simulink model "Model_InterpretationEngine64"  (R2022b)
settings: Solver=FixedStepDiscrete  StartTime=0.0  StopTime=5  RelTol=1e-3  EnableMultiTasking=on
InitFcn:
  | % Initialize model
  | ModelSettings=BTConfig.GetModelSettings();
  | 
  | ModelSettings.Validate();
  | 
  | ModelInit;
  | 
  | 
  | % load library data
  | GainLibrary_data;
  | % Load saved values from partition process
  | CapturedConstMask.LoadMapFromFile(bdroot)
  | % Load saved values from partition process
  | TSP_Mask.LoadMapFromFile(bdroot)
StartFcn:
  | % make sure all the simulated RTC requests are found
  | %RTC_SIM_OBJ.ValidateREQs();
undefined symbols (not defined in the file or in its folder): NumHFRefBPF, NumHFRefLPF
libraries: StateVar x112, TSP x56, FeaturePath x24
(part 3 of 5)

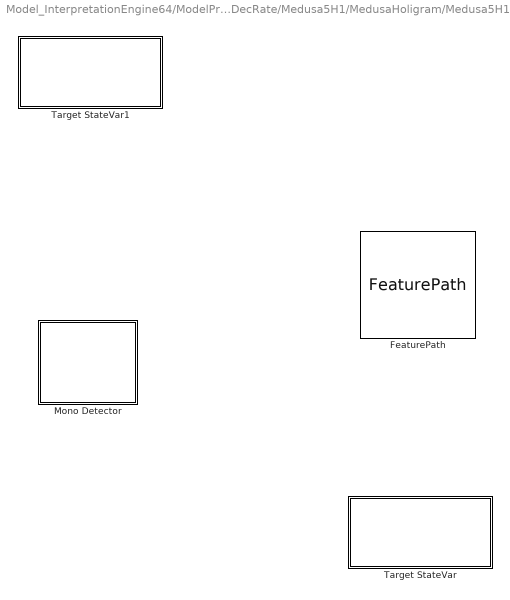
== system Model_InterpretationEngine64/ModelPreAmp/DecRate/Medusa5H1/MedusaHoligram/Medusa5H1 Part 2/Mono Detector ==
  FeaturePath : FeaturePath/FeaturePath  FeatureName=MonoDetector  IsGroup=off  GroupNumber=-1  IsModule=off  TriggerInit=[680 129 795 236]
      settings: SourceProductName=Bose Talaria
  Mono Detector : Subsystem
  Target StateVar : Subsystem  mask(Talaria Target State Variable){TriggerInit=[670 396 810 464], TspName=IsStereo, StateName=IsStereo, UseSameName=on, IfdefMacro=[]}
      mask prompts: TriggerInit "Hidden: MoveFcn redraw"; TspName "Name:"; StateName "Name of StateVar:"; UseSameName "Use same name for state variable and TSP"; IfdefMacro "Additional #ifdef macro to enable trigger capture:"
      mask help: The TargetStateVar block encapsultes a Target State Probe (TSP), a State Variable, and a Trivial Interpretation between them.
      mask init:
      | [ok,tspPath,activeStatePath] = TargetStateVarMask.Init(gcbh);
      settings: MoveFcn=TargetStateVarMask.CB_TriggerInit(gcbh);
      mask Help: See help for StateVar and TSP blocks
      mask Callback TriggerInit: TargetStateVarMask.CB_TriggerInit(gcbh);
      mask TypeOptions TspName: TSP/TspName
      mask TypeOptions StateName: StateVar/StateName
      mask Callback UseSameName: TargetStateVarMask.CB_UseSameName(gcbh);
      mask TypeOptions IfdefMacro: TSP/IfdefMacro
      mask DialogControl AdvancedPanel Prompt: Advanced
      mask DialogControl ConvertToFullInterpretation Prompt: Irreversible conversion to full interpretation
      mask DialogControl ConvertToFullInterpretation Callback: TargetStateVarMask.CB_ConvertToFullInterpretation(gcbh);
      mask DialogControl ErrorContainer Prompt: Error Messages
      mask DialogControl ErrorText Prompt: The interpreted StateVar value is not yet available
      mask DialogControl TspPathText Prompt: TSP: Current parameter name: [PreAmpMedusaMonoDetectorIsStereo]
      mask Display:
      | % retrieve icon definition
      | [path,w,h] = TargetStateVarMask.Icon();
      | 
      | % retrieve the block's pixel size
      | pos = get(gcbh,'position');
      | bw = pos(3) - pos(1);
      | bh = pos(4) - pos(2);
      | 
      | % draw centered icon
      | xAdj = bw/2 - w/2 + 5;
      | yAdj = bh/2 - h/2 + 4;
      | for i=1:length(path)
      | 	patch(path(i).x+xAdj, path(i).y+yAdj, path(i).rgb);
      | end
      | 
      | % show the top name or an X
      | if (exist('ok','var') && ok)
      | 	text(bw*0.5, bh*0.2, tspPath, 'horizontalAlignment', 'center');
      | 	patch(0,0,[1 1 1]);
      | 	patch(bw,bh,[1 1 1]);
      | else
      | 	tx=bw*0.03;
      | 	ty=bh*0.03;
      | 	patch([0 tx bw bw-tx], [ty 0 bh-ty bh], [1 0 0]);
      | 	patch([0 bw-tx bw tx], [bh-ty 0 ty bh], [1 0 0]);
      | end
  Target StateVar1 : Subsystem  mask(Talaria Target State Variable){TriggerInit=[340 131 480 199], TspName=IsActive, StateName=IsActive, UseSameName=on, IfdefMacro=[]}
      mask prompts: TriggerInit "Hidden: MoveFcn redraw"; TspName "Name:"; StateName "Name of StateVar:"; UseSameName "Use same name for state variable and TSP"; IfdefMacro "Additional #ifdef macro to enable trigger capture:"
      mask help: The TargetStateVar block encapsultes a Target State Probe (TSP), a State Variable, and a Trivial Interpretation between them.
      mask init:
      | [ok,tspPath,activeStatePath] = TargetStateVarMask.Init(gcbh);
      settings: MoveFcn=TargetStateVarMask.CB_TriggerInit(gcbh);
      mask Help: See help for StateVar and TSP blocks
      mask Callback TriggerInit: TargetStateVarMask.CB_TriggerInit(gcbh);
      mask TypeOptions TspName: TSP/TspName
      mask TypeOptions StateName: StateVar/StateName
      mask Callback UseSameName: TargetStateVarMask.CB_UseSameName(gcbh);
      mask TypeOptions IfdefMacro: TSP/IfdefMacro
      mask DialogControl AdvancedPanel Prompt: Advanced
      mask DialogControl ConvertToFullInterpretation Prompt: Irreversible conversion to full interpretation
      mask DialogControl ConvertToFullInterpretation Callback: TargetStateVarMask.CB_ConvertToFullInterpretation(gcbh);
      mask DialogControl ErrorContainer Prompt: Error Messages
      mask DialogControl ErrorText Prompt: The interpreted StateVar value is not yet available
      mask DialogControl TspPathText Prompt: TSP: Current parameter name: [PreAmpMedusaMonoDetectorIsActive]
      mask Display:
      | % retrieve icon definition
      | [path,w,h] = TargetStateVarMask.Icon();
      | 
      | % retrieve the block's pixel size
      | pos = get(gcbh,'position');
      | bw = pos(3) - pos(1);
      | bh = pos(4) - pos(2);
      | 
      | % draw centered icon
      | xAdj = bw/2 - w/2 + 5;
      | yAdj = bh/2 - h/2 + 4;
      | for i=1:length(path)
      | 	patch(path(i).x+xAdj, path(i).y+yAdj, path(i).rgb);
      | end
      | 
      | % show the top name or an X
      | if (exist('ok','var') && ok)
      | 	text(bw*0.5, bh*0.2, tspPath, 'horizontalAlignment', 'center');
      | 	patch(0,0,[1 1 1]);
      | 	patch(bw,bh,[1 1 1]);
      | else
      | 	tx=bw*0.03;
      | 	ty=bh*0.03;
      | 	patch([0 tx bw bw-tx], [ty 0 bh-ty bh], [1 0 0]);
      | 	patch([0 bw-tx bw tx], [bh-ty 0 ty bh], [1 0 0]);
      | end

== system Model_InterpretationEngine64/NEAR/Near1p1/VolumeMute/VolMuteCh1/Ann1NonEntGainCalc/boost ==
  Target StateVar : Subsystem  mask(Talaria Target State Variable){TriggerInit=[655 408 850 472], TspName=GetNonEntBoostLeveldB, StateName=GetNonEntBoostLeveldB, UseSameName=on, IfdefMacro=[]}
      mask prompts: TriggerInit "Hidden: MoveFcn redraw"; TspName "Name:"; StateName "Name of StateVar:"; UseSameName "Use same name for state variable and TSP"; IfdefMacro "Additional #ifdef macro to enable trigger capture:"
      mask help: The TargetStateVar block encapsultes a Target State Probe (TSP), a State Variable, and a Trivial Interpretation between them.
      mask init:
      | [ok,tspPath,activeStatePath] = TargetStateVarMask.Init(gcbh);
      settings: MoveFcn=TargetStateVarMask.CB_TriggerInit(gcbh);
      mask Help: See help for StateVar and TSP blocks
      mask Callback TriggerInit: TargetStateVarMask.CB_TriggerInit(gcbh);
      mask TypeOptions TspName: TSP/TspName
      mask TypeOptions StateName: StateVar/StateName
      mask Callback UseSameName: TargetStateVarMask.CB_UseSameName(gcbh);
      mask TypeOptions IfdefMacro: TSP/IfdefMacro
      mask DialogControl AdvancedPanel Prompt: Advanced
      mask DialogControl ConvertToFullInterpretation Prompt: Irreversible conversion to full interpretation
      mask DialogControl ConvertToFullInterpretation Callback: TargetStateVarMask.CB_ConvertToFullInterpretation(gcbh);
      mask DialogControl ErrorContainer Prompt: Error Messages
      mask DialogControl ErrorText Prompt: The interpreted StateVar value is not yet available
      mask DialogControl TspPathText Prompt: TSP: Current parameter name: [NearAnn1Ann1NonEntGainCalcGetNonEntBoostLeveldB]
      mask Display:
      | % retrieve icon definition
      | [path,w,h] = TargetStateVarMask.Icon();
      | 
      | % retrieve the block's pixel size
      | pos = get(gcbh,'position');
      | bw = pos(3) - pos(1);
      | bh = pos(4) - pos(2);
      | 
      | % draw centered icon
      | xAdj = bw/2 - w/2 + 5;
      | yAdj = bh/2 - h/2 + 4;
      | for i=1:length(path)
      | 	patch(path(i).x+xAdj, path(i).y+yAdj, path(i).rgb);
      | end
      | 
      | % show the top name or an X
      | if (exist('ok','var') && ok)
      | 	text(bw*0.5, bh*0.2, tspPath, 'horizontalAlignment', 'center');
      | 	patch(0,0,[1 1 1]);
      | 	patch(bw,bh,[1 1 1]);
      | else
      | 	tx=bw*0.03;
      | 	ty=bh*0.03;
      | 	patch([0 tx bw bw-tx], [ty 0 bh-ty bh], [1 0 0]);
      | 	patch([0 bw-tx bw tx], [bh-ty 0 ty bh], [1 0 0]);
      | end

== system Model_InterpretationEngine64/NEAR/Near1p1/VolumeMute/VolMuteCh2/Ann2NonEntGainCalc/boost ==
  Target StateVar : Subsystem  mask(Talaria Target State Variable){TriggerInit=[655 408 850 472], TspName=GetNonEntBoostLeveldB, StateName=GetNonEntBoostLeveldB, UseSameName=on, IfdefMacro=[]}
      mask prompts: TriggerInit "Hidden: MoveFcn redraw"; TspName "Name:"; StateName "Name of StateVar:"; UseSameName "Use same name for state variable and TSP"; IfdefMacro "Additional #ifdef macro to enable trigger capture:"
      mask help: The TargetStateVar block encapsultes a Target State Probe (TSP), a State Variable, and a Trivial Interpretation between them.
      mask init:
      | [ok,tspPath,activeStatePath] = TargetStateVarMask.Init(gcbh);
      settings: MoveFcn=TargetStateVarMask.CB_TriggerInit(gcbh);
      mask Help: See help for StateVar and TSP blocks
      mask Callback TriggerInit: TargetStateVarMask.CB_TriggerInit(gcbh);
      mask TypeOptions TspName: TSP/TspName
      mask TypeOptions StateName: StateVar/StateName
      mask Callback UseSameName: TargetStateVarMask.CB_UseSameName(gcbh);
      mask TypeOptions IfdefMacro: TSP/IfdefMacro
      mask DialogControl AdvancedPanel Prompt: Advanced
      mask DialogControl ConvertToFullInterpretation Prompt: Irreversible conversion to full interpretation
      mask DialogControl ConvertToFullInterpretation Callback: TargetStateVarMask.CB_ConvertToFullInterpretation(gcbh);
      mask DialogControl ErrorContainer Prompt: Error Messages
      mask DialogControl ErrorText Prompt: The interpreted StateVar value is not yet available
      mask DialogControl TspPathText Prompt: TSP: Current parameter name: [NearAnn2Ann2NonEntGainCalcGetNonEntBoostLeveldB]
      mask Display:
      | % retrieve icon definition
      | [path,w,h] = TargetStateVarMask.Icon();
      | 
      | % retrieve the block's pixel size
      | pos = get(gcbh,'position');
      | bw = pos(3) - pos(1);
      | bh = pos(4) - pos(2);
      | 
      | % draw centered icon
      | xAdj = bw/2 - w/2 + 5;
      | yAdj = bh/2 - h/2 + 4;
      | for i=1:length(path)
      | 	patch(path(i).x+xAdj, path(i).y+yAdj, path(i).rgb);
      | end
      | 
      | % show the top name or an X
      | if (exist('ok','var') && ok)
      | 	text(bw*0.5, bh*0.2, tspPath, 'horizontalAlignment', 'center');
      | 	patch(0,0,[1 1 1]);
      | 	patch(bw,bh,[1 1 1]);
      | else
      | 	tx=bw*0.03;
      | 	ty=bh*0.03;
      | 	patch([0 tx bw bw-tx], [ty 0 bh-ty bh], [1 0 0]);
      | 	patch([0 bw-tx bw tx], [bh-ty 0 ty bh], [1 0 0]);
      | end

== system Model_InterpretationEngine64/NEAR/Near1p1/VolumeMute/VolMuteCh3/Ann3NonEntGainCalc/boost ==
  Target StateVar : Subsystem  mask(Talaria Target State Variable){TriggerInit=[655 408 850 472], TspName=GetNonEntBoostLeveldB, StateName=GetNonEntBoostLeveldB, UseSameName=on, IfdefMacro=[]}
      mask prompts: TriggerInit "Hidden: MoveFcn redraw"; TspName "Name:"; StateName "Name of StateVar:"; UseSameName "Use same name for state variable and TSP"; IfdefMacro "Additional #ifdef macro to enable trigger capture:"
      mask help: The TargetStateVar block encapsultes a Target State Probe (TSP), a State Variable, and a Trivial Interpretation between them.
      mask init:
      | [ok,tspPath,activeStatePath] = TargetStateVarMask.Init(gcbh);
      settings: MoveFcn=TargetStateVarMask.CB_TriggerInit(gcbh);
      mask Help: See help for StateVar and TSP blocks
      mask Callback TriggerInit: TargetStateVarMask.CB_TriggerInit(gcbh);
      mask TypeOptions TspName: TSP/TspName
      mask TypeOptions StateName: StateVar/StateName
      mask Callback UseSameName: TargetStateVarMask.CB_UseSameName(gcbh);
      mask TypeOptions IfdefMacro: TSP/IfdefMacro
      mask DialogControl AdvancedPanel Prompt: Advanced
      mask DialogControl ConvertToFullInterpretation Prompt: Irreversible conversion to full interpretation
      mask DialogControl ConvertToFullInterpretation Callback: TargetStateVarMask.CB_ConvertToFullInterpretation(gcbh);
      mask DialogControl ErrorContainer Prompt: Error Messages
      mask DialogControl ErrorText Prompt: The interpreted StateVar value is not yet available
      mask DialogControl TspPathText Prompt: TSP: Current parameter name: [NearAnn3Ann3NonEntGainCalcGetNonEntBoostLeveldB]
      mask Display:
      | % retrieve icon definition
      | [path,w,h] = TargetStateVarMask.Icon();
      | 
      | % retrieve the block's pixel size
      | pos = get(gcbh,'position');
      | bw = pos(3) - pos(1);
      | bh = pos(4) - pos(2);
      | 
      | % draw centered icon
      | xAdj = bw/2 - w/2 + 5;
      | yAdj = bh/2 - h/2 + 4;
      | for i=1:length(path)
      | 	patch(path(i).x+xAdj, path(i).y+yAdj, path(i).rgb);
      | end
      | 
      | % show the top name or an X
      | if (exist('ok','var') && ok)
      | 	text(bw*0.5, bh*0.2, tspPath, 'horizontalAlignment', 'center');
      | 	patch(0,0,[1 1 1]);
      | 	patch(bw,bh,[1 1 1]);
      | else
      | 	tx=bw*0.03;
      | 	ty=bh*0.03;
      | 	patch([0 tx bw bw-tx], [ty 0 bh-ty bh], [1 0 0]);
      | 	patch([0 bw-tx bw tx], [bh-ty 0 ty bh], [1 0 0]);
      | end

== system Model_InterpretationEngine64/NEAR/Near1p1/VolumeMute/VolMuteCh4/Ann4NonEntGainCalc/boost ==
  Target StateVar : Subsystem  mask(Talaria Target State Variable){TriggerInit=[655 408 850 472], TspName=GetNonEntBoostLeveldB, StateName=GetNonEntBoostLeveldB, UseSameName=on, IfdefMacro=[]}
      mask prompts: TriggerInit "Hidden: MoveFcn redraw"; TspName "Name:"; StateName "Name of StateVar:"; UseSameName "Use same name for state variable and TSP"; IfdefMacro "Additional #ifdef macro to enable trigger capture:"
      mask help: The TargetStateVar block encapsultes a Target State Probe (TSP), a State Variable, and a Trivial Interpretation between them.
      mask init:
      | [ok,tspPath,activeStatePath] = TargetStateVarMask.Init(gcbh);
      settings: MoveFcn=TargetStateVarMask.CB_TriggerInit(gcbh);
      mask Help: See help for StateVar and TSP blocks
      mask Callback TriggerInit: TargetStateVarMask.CB_TriggerInit(gcbh);
      mask TypeOptions TspName: TSP/TspName
      mask TypeOptions StateName: StateVar/StateName
      mask Callback UseSameName: TargetStateVarMask.CB_UseSameName(gcbh);
      mask TypeOptions IfdefMacro: TSP/IfdefMacro
      mask DialogControl AdvancedPanel Prompt: Advanced
      mask DialogControl ConvertToFullInterpretation Prompt: Irreversible conversion to full interpretation
      mask DialogControl ConvertToFullInterpretation Callback: TargetStateVarMask.CB_ConvertToFullInterpretation(gcbh);
      mask DialogControl ErrorContainer Prompt: Error Messages
      mask DialogControl ErrorText Prompt: The interpreted StateVar value is not yet available
      mask DialogControl TspPathText Prompt: TSP: Current parameter name: [NearAnn4Ann4NonEntGainCalcGetNonEntBoostLeveldB]
      mask Display:
      | % retrieve icon definition
      | [path,w,h] = TargetStateVarMask.Icon();
      | 
      | % retrieve the block's pixel size
      | pos = get(gcbh,'position');
      | bw = pos(3) - pos(1);
      | bh = pos(4) - pos(2);
      | 
      | % draw centered icon
      | xAdj = bw/2 - w/2 + 5;
      | yAdj = bh/2 - h/2 + 4;
      | for i=1:length(path)
      | 	patch(path(i).x+xAdj, path(i).y+yAdj, path(i).rgb);
      | end
      | 
      | % show the top name or an X
      | if (exist('ok','var') && ok)
      | 	text(bw*0.5, bh*0.2, tspPath, 'horizontalAlignment', 'center');
      | 	patch(0,0,[1 1 1]);
      | 	patch(bw,bh,[1 1 1]);
      | else
      | 	tx=bw*0.03;
      | 	ty=bh*0.03;
      | 	patch([0 tx bw bw-tx], [ty 0 bh-ty bh], [1 0 0]);
      | 	patch([0 bw-tx bw tx], [bh-ty 0 ty bh], [1 0 0]);
      | end

== system Model_InterpretationEngine64/PostProcess/PostProcess/EnergyLimiter/EnergyLimiter1/EnergyRunningAvg /Target StateVar ==
  StateVar : StateVar/StateVar  TriggerInit=[490 139 605 201]  StateName=ComputedEnergy
      settings: SourceProductName=Bose Talaria
  TSP : TSP/TSP  TriggerInit=[110 134 215 206]  TspName=ComputedEnergy  IfDefMacro=IfdefMacro  Role=Automatic
      settings: SourceProductName=Bose Talaria
  TrivialInterpretation : StateVar/TrivialInterpretation  TriggerInit=[330 148 380 192]
      settings: SourceProductName=Bose Talaria
  wires:
  TrivialInterpretation/1 -> StateVar/1
  TSP/1 -> TrivialInterpretation/1

== system Model_InterpretationEngine64/PostProcess/PostProcess/EnergyLimiter/EnergyLimiter1/EnergyRunningAvg /Target StateVar1 ==
  StateVar : StateVar/StateVar  TriggerInit=[490 139 605 201]  StateName=CurGain
      settings: SourceProductName=Bose Talaria
  TSP : TSP/TSP  TriggerInit=[110 134 215 206]  TspName=CurGain  IfDefMacro=IfdefMacro  Role=Automatic
      settings: SourceProductName=Bose Talaria
  TrivialInterpretation : StateVar/TrivialInterpretation  TriggerInit=[330 148 380 192]
      settings: SourceProductName=Bose Talaria
  wires:
  TrivialInterpretation/1 -> StateVar/1
  TSP/1 -> TrivialInterpretation/1

== system Model_InterpretationEngine64/PostProcess/PostProcess/EnergyLimiter/EnergyLimiter1/EnergyRunningAvg /Target StateVar2 ==
  StateVar : StateVar/StateVar  TriggerInit=[490 139 605 201]  StateName=EnergyThreshold
      settings: SourceProductName=Bose Talaria
  TSP : TSP/TSP  TriggerInit=[110 134 215 206]  TspName=EnergyThreshold  IfDefMacro=IfdefMacro  Role=Automatic
      settings: SourceProductName=Bose Talaria
  TrivialInterpretation : StateVar/TrivialInterpretation  TriggerInit=[330 148 380 192]
      settings: SourceProductName=Bose Talaria
  wires:
  TrivialInterpretation/1 -> StateVar/1
  TSP/1 -> TrivialInterpretation/1

== system Model_InterpretationEngine64/PostProcess/PostProcess/EnergyLimiter/EnergyLimiter1/EnergyRunningAvg /Target StateVar3 ==
  StateVar : StateVar/StateVar  TriggerInit=[490 139 605 201]  StateName=CurState
      settings: SourceProductName=Bose Talaria
  TSP : TSP/TSP  TriggerInit=[110 134 215 206]  TspName=CurState  IfDefMacro=IfdefMacro  Role=Automatic
      settings: SourceProductName=Bose Talaria
  TrivialInterpretation : StateVar/TrivialInterpretation  TriggerInit=[330 148 380 192]
      settings: SourceProductName=Bose Talaria
  wires:
  TrivialInterpretation/1 -> StateVar/1
  TSP/1 -> TrivialInterpretation/1

== system Model_InterpretationEngine64/PostProcess/PostProcess/EnergyLimiter/EnergyLimiter1/EnergyRunningAvg /Target StateVar4 ==
  StateVar : StateVar/StateVar  TriggerInit=[490 139 605 201]  StateName=EnableFlag
      settings: SourceProductName=Bose Talaria
  TSP : TSP/TSP  TriggerInit=[110 134 215 206]  TspName=EnableFlag  IfDefMacro=IfdefMacro  Role=Automatic
      settings: SourceProductName=Bose Talaria
  TrivialInterpretation : StateVar/TrivialInterpretation  TriggerInit=[330 148 380 192]
      settings: SourceProductName=Bose Talaria
  wires:
  TrivialInterpretation/1 -> StateVar/1
  TSP/1 -> TrivialInterpretation/1

== system Model_InterpretationEngine64/ModelPreAmp/DecRate/AudioPilot35/Audiopilot_3_5/GainCalculation/Monitoring/AudiopilotBassBoost ==
  StateVar : StateVar/StateVar  TriggerInit=[490 139 605 201]  StateName=AudiopilotBassBoostDb
      settings: SourceProductName=Bose Talaria
  TSP : TSP/TSP  TriggerInit=[110 134 215 206]  TspName=AudiopilotBassBoostDb  IfDefMacro=IfdefMacro  Role=Automatic
      settings: SourceProductName=Bose Talaria
  TrivialInterpretation : StateVar/TrivialInterpretation  TriggerInit=[330 148 380 192]
      settings: SourceProductName=Bose Talaria
  wires:
  TSP/1 -> TrivialInterpretation/1
  TrivialInterpretation/1 -> StateVar/1

== system Model_InterpretationEngine64/ModelPreAmp/DecRate/AudioPilot35/Audiopilot_3_5/GainCalculation/Monitoring/AudiopilotMidrangeBoost ==
  StateVar : StateVar/StateVar  TriggerInit=[490 139 605 201]  StateName=AudiopilotMidrangeBoostDb
      settings: SourceProductName=Bose Talaria
  TSP : TSP/TSP  TriggerInit=[110 134 215 206]  TspName=AudiopilotMidrangeBoostDb  IfDefMacro=IfdefMacro  Role=Automatic
      settings: SourceProductName=Bose Talaria
  TrivialInterpretation : StateVar/TrivialInterpretation  TriggerInit=[330 148 380 192]
      settings: SourceProductName=Bose Talaria
  wires:
  TSP/1 -> TrivialInterpretation/1
  TrivialInterpretation/1 -> StateVar/1

== system Model_InterpretationEngine64/ModelPreAmp/DecRate/AudioPilot35/Audiopilot_3_5/GainCalculation/Monitoring/AudiopilotTrebleBoost ==
  StateVar : StateVar/StateVar  TriggerInit=[490 139 605 201]  StateName=AudiopilotTrebleBoostDb
      settings: SourceProductName=Bose Talaria
  TSP : TSP/TSP  TriggerInit=[110 134 215 206]  TspName=AudiopilotTrebleBoostDb  IfDefMacro=IfdefMacro  Role=Automatic
      settings: SourceProductName=Bose Talaria
  TrivialInterpretation : StateVar/TrivialInterpretation  TriggerInit=[330 148 380 192]
      settings: SourceProductName=Bose Talaria
  wires:
  TSP/1 -> TrivialInterpretation/1
  TrivialInterpretation/1 -> StateVar/1

== system Model_InterpretationEngine64/ModelPreAmp/DecRate/AudioPilot35/Audiopilot_3_5/GainCalculation/Monitoring/DyneqBassBoost ==
  StateVar : StateVar/StateVar  TriggerInit=[490 139 605 201]  StateName=DyneqBassBoostDb
      settings: SourceProductName=Bose Talaria
  TSP : TSP/TSP  TriggerInit=[110 134 215 206]  TspName=DyneqBassBoostDb  IfDefMacro=IfdefMacro  Role=Automatic
      settings: SourceProductName=Bose Talaria
  TrivialInterpretation : StateVar/TrivialInterpretation  TriggerInit=[330 148 380 192]
      settings: SourceProductName=Bose Talaria
  wires:
  TSP/1 -> TrivialInterpretation/1
  TrivialInterpretation/1 -> StateVar/1

== system Model_InterpretationEngine64/ModelPreAmp/DecRate/AudioPilot35/Audiopilot_3_5/GainCalculation/Monitoring/HfNoise ==
  StateVar : StateVar/StateVar  TriggerInit=[490 139 605 201]  StateName=HfNoiseDbspl
      settings: SourceProductName=Bose Talaria
  TSP : TSP/TSP  TriggerInit=[110 134 215 206]  TspName=HfNoiseDbspl  IfDefMacro=IfdefMacro  Role=Automatic
      settings: SourceProductName=Bose Talaria
  TrivialInterpretation : StateVar/TrivialInterpretation  TriggerInit=[330 148 380 192]
      settings: SourceProductName=Bose Talaria
  wires:
  TSP/1 -> TrivialInterpretation/1
  TrivialInterpretation/1 -> StateVar/1

== system Model_InterpretationEngine64/ModelPreAmp/DecRate/AudioPilot35/Audiopilot_3_5/GainCalculation/Monitoring/IgnoreMic ==
  StateVar : StateVar/StateVar  TriggerInit=[490 139 605 201]  StateName=IgnoreMicFlag
      settings: SourceProductName=Bose Talaria
  TSP : TSP/TSP  TriggerInit=[110 134 215 206]  TspName=IgnoreMicFlag  IfDefMacro=IfdefMacro  Role=Automatic
      settings: SourceProductName=Bose Talaria
  TrivialInterpretation : StateVar/TrivialInterpretation  TriggerInit=[330 148 380 192]
      settings: SourceProductName=Bose Talaria
  wires:
  TSP/1 -> TrivialInterpretation/1
  TrivialInterpretation/1 -> StateVar/1

== system Model_InterpretationEngine64/ModelPreAmp/DecRate/AudioPilot35/Audiopilot_3_5/GainCalculation/Monitoring/LfNoise ==
  StateVar : StateVar/StateVar  TriggerInit=[490 139 605 201]  StateName=LfNoiseDbspl
      settings: SourceProductName=Bose Talaria
  TSP : TSP/TSP  TriggerInit=[110 134 215 206]  TspName=LfNoiseDbspl  IfDefMacro=IfdefMacro  Role=Automatic
      settings: SourceProductName=Bose Talaria
  TrivialInterpretation : StateVar/TrivialInterpretation  TriggerInit=[330 148 380 192]
      settings: SourceProductName=Bose Talaria
  wires:
  TSP/1 -> TrivialInterpretation/1
  TrivialInterpretation/1 -> StateVar/1

== system Model_InterpretationEngine64/ModelPreAmp/DecRate/AudioPilot35/Audiopilot_3_5/GainCalculation/Monitoring/NoiseRatio ==
  StateVar : StateVar/StateVar  TriggerInit=[490 139 605 201]  StateName=NoiseRatio
      settings: SourceProductName=Bose Talaria
  TSP : TSP/TSP  TriggerInit=[110 134 215 206]  TspName=NoiseRatio  IfDefMacro=IfdefMacro  Role=Automatic
      settings: SourceProductName=Bose Talaria
  TrivialInterpretation : StateVar/TrivialInterpretation  TriggerInit=[330 148 380 192]
      settings: SourceProductName=Bose Talaria
  wires:
  TSP/1 -> TrivialInterpretation/1
  TrivialInterpretation/1 -> StateVar/1

== system Model_InterpretationEngine64/ModelPreAmp/DecRate/AudioPilot35/Audiopilot_3_5/GainCalculation/Monitoring/TotalBassBoost ==
  StateVar : StateVar/StateVar  TriggerInit=[490 139 605 201]  StateName=TotalBassBoostDb
      settings: SourceProductName=Bose Talaria
  TSP : TSP/TSP  TriggerInit=[110 134 215 206]  TspName=TotalBassBoostDb  IfDefMacro=IfdefMacro  Role=Automatic
      settings: SourceProductName=Bose Talaria
  TrivialInterpretation : StateVar/TrivialInterpretation  TriggerInit=[330 148 380 192]
      settings: SourceProductName=Bose Talaria
  wires:
  TSP/1 -> TrivialInterpretation/1
  TrivialInterpretation/1 -> StateVar/1

== system Model_InterpretationEngine64/ModelPreAmp/DecRate/AudioPilot35/Audiopilot_3_5/GainCalculation/Monitoring/WbNoise ==
  StateVar : StateVar/StateVar  TriggerInit=[490 139 605 201]  StateName=WbNoiseDbspl
      settings: SourceProductName=Bose Talaria
  TSP : TSP/TSP  TriggerInit=[110 134 215 206]  TspName=WbNoiseDbspl  IfDefMacro=IfdefMacro  Role=Automatic
      settings: SourceProductName=Bose Talaria
  TrivialInterpretation : StateVar/TrivialInterpretation  TriggerInit=[330 148 380 192]
      settings: SourceProductName=Bose Talaria
  wires:
  TSP/1 -> TrivialInterpretation/1
  TrivialInterpretation/1 -> StateVar/1

== system Model_InterpretationEngine64/ModelPreAmp/DecRate/AudioPilot35/Audiopilot_3_5/GainCalculation/RampedEnable/audiopilot boost gain ==
  StateVar : StateVar/StateVar  TriggerInit=[490 139 605 201]  StateName=AudiopilotBoostGain
      settings: SourceProductName=Bose Talaria
  TSP : TSP/TSP  TriggerInit=[110 134 215 206]  TspName=AudiopilotBoostGain  IfDefMacro=IfdefMacro  Role=Automatic
      settings: SourceProductName=Bose Talaria
  TrivialInterpretation : StateVar/TrivialInterpretation  TriggerInit=[330 148 380 192]
      settings: SourceProductName=Bose Talaria
  wires:
  TSP/1 -> TrivialInterpretation/1
  TrivialInterpretation/1 -> StateVar/1

== system Model_InterpretationEngine64/ModelPreAmp/DecRate/AudioPilot35/Audiopilot_3_5/GainCalculation/RampedEnable/dyneq boost gain ==
  StateVar : StateVar/StateVar  TriggerInit=[490 139 605 201]  StateName=DyneqBoostGain
      settings: SourceProductName=Bose Talaria
  TSP : TSP/TSP  TriggerInit=[110 134 215 206]  TspName=DyneqBoostGain  IfDefMacro=IfdefMacro  Role=Automatic
      settings: SourceProductName=Bose Talaria
  TrivialInterpretation : StateVar/TrivialInterpretation  TriggerInit=[330 148 380 192]
      settings: SourceProductName=Bose Talaria
  wires:
  TSP/1 -> TrivialInterpretation/1
  TrivialInterpretation/1 -> StateVar/1

== system Model_InterpretationEngine64/ModelPreAmp/DecRate/AudioPilot35/Audiopilot_3_5/NoiseEstimationVariant/RegularNoiseEstimation/HFNoiseEstimatorCoh ==
  FeaturePath : FeaturePath/FeaturePath  FeatureName=HfNoise  IsGroup=off  GroupNumber=-1  IsModule=off  TriggerInit=[360 -186 485 -69]
      settings: SourceProductName=Bose Talaria
  "HfNoiseMusicSeparation " : Subsystem
  PostProcessing : Subsystem

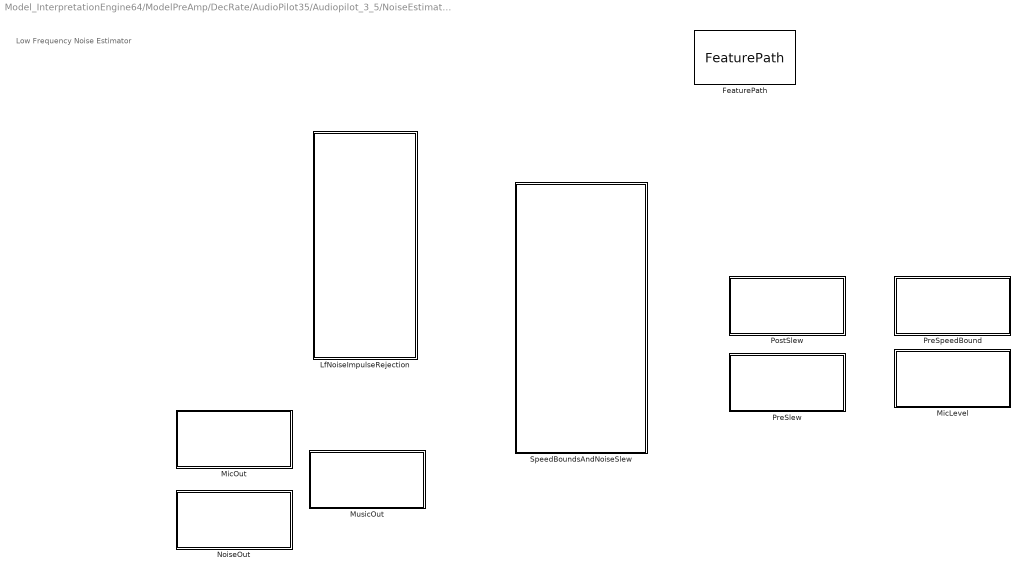
== system Model_InterpretationEngine64/ModelPreAmp/DecRate/AudioPilot35/Audiopilot_3_5/NoiseEstimationVariant/RegularNoiseEstimation/LFNoiseEstimatorCoh ==
  note: Low Frequency Noise Estimator
  FeaturePath : FeaturePath/FeaturePath  FeatureName=LfNoise  IsGroup=off  GroupNumber=-1  IsModule=off  TriggerInit=[975 -106 1100 -39]
      settings: SourceProductName=Bose Talaria
  LfNoiseImpulseRejection : Subsystem
  MicLevel : Subsystem  mask(Talaria Target State Variable){TriggerInit=[1225 291 1365 359], TspName=MicLevel, StateName=MicLevel, UseSameName=on, IfdefMacro=[]}
      mask prompts: TriggerInit "Hidden: MoveFcn redraw"; TspName "Name:"; StateName "Name of StateVar:"; UseSameName "Use same name for state variable and TSP"; IfdefMacro "Additional #ifdef macro to enable trigger capture:"
      mask help: The TargetStateVar block encapsultes a Target State Probe (TSP), a State Variable, and a Trivial Interpretation between them.
      mask init:
      | [ok,tspPath,activeStatePath] = TargetStateVarMask.Init(gcbh);
      settings: MoveFcn=TargetStateVarMask.CB_TriggerInit(gcbh);
      mask Help: See help for StateVar and TSP blocks
      mask Callback TriggerInit: TargetStateVarMask.CB_TriggerInit(gcbh);
      mask TypeOptions TspName: TSP/TspName
      mask TypeOptions StateName: StateVar/StateName
      mask Callback UseSameName: TargetStateVarMask.CB_UseSameName(gcbh);
      mask TypeOptions IfdefMacro: TSP/IfdefMacro
      mask DialogControl AdvancedPanel Prompt: Advanced
      mask DialogControl ConvertToFullInterpretation Prompt: Irreversible conversion to full interpretation
      mask DialogControl ConvertToFullInterpretation Callback: TargetStateVarMask.CB_ConvertToFullInterpretation(gcbh);
      mask DialogControl ErrorContainer Prompt: Error Messages
      mask DialogControl ErrorText Prompt: The interpreted StateVar value is not yet available
      mask DialogControl TspPathText Prompt: TSP: Current parameter name: [AudiopilotLfNoiseMicLevel]
      mask Display:
      | % retrieve icon definition
      | [path,w,h] = TargetStateVarMask.Icon();
      | 
      | % retrieve the block's pixel size
      | pos = get(gcbh,'position');
      | bw = pos(3) - pos(1);
      | bh = pos(4) - pos(2);
      | 
      | % draw centered icon
      | xAdj = bw/2 - w/2 + 5;
      | yAdj = bh/2 - h/2 + 4;
      | for i=1:length(path)
      | 	patch(path(i).x+xAdj, path(i).y+yAdj, path(i).rgb);
      | end
      | 
      | % show the top name or an X
      | if (exist('ok','var') && ok)
      | 	text(bw*0.5, bh*0.2, tspPath, 'horizontalAlignment', 'center');
      | 	patch(0,0,[1 1 1]);
      | 	patch(bw,bh,[1 1 1]);
      | else
      | 	tx=bw*0.03;
      | 	ty=bh*0.03;
      | 	patch([0 tx bw bw-tx], [ty 0 bh-ty bh], [1 0 0]);
      | 	patch([0 bw-tx bw tx], [bh-ty 0 ty bh], [1 0 0]);
      | end
  MicOut : Subsystem  mask(Talaria Target State Variable){TriggerInit=[335 366 475 434], TspName=MicOut, StateName=MicOut, UseSameName=on, IfdefMacro=[]}
      mask prompts: TriggerInit "Hidden: MoveFcn redraw"; TspName "Name:"; StateName "Name of StateVar:"; UseSameName "Use same name for state variable and TSP"; IfdefMacro "Additional #ifdef macro to enable trigger capture:"
      mask help: The TargetStateVar block encapsultes a Target State Probe (TSP), a State Variable, and a Trivial Interpretation between them.
      mask init:
      | [ok,tspPath,activeStatePath] = TargetStateVarMask.Init(gcbh);
      settings: MoveFcn=TargetStateVarMask.CB_TriggerInit(gcbh);
      mask Help: See help for StateVar and TSP blocks
      mask Callback TriggerInit: TargetStateVarMask.CB_TriggerInit(gcbh);
      mask TypeOptions TspName: TSP/TspName
      mask TypeOptions StateName: StateVar/StateName
      mask Callback UseSameName: TargetStateVarMask.CB_UseSameName(gcbh);
      mask TypeOptions IfdefMacro: TSP/IfdefMacro
      mask DialogControl AdvancedPanel Prompt: Advanced
      mask DialogControl ConvertToFullInterpretation Prompt: Irreversible conversion to full interpretation
      mask DialogControl ConvertToFullInterpretation Callback: TargetStateVarMask.CB_ConvertToFullInterpretation(gcbh);
      mask DialogControl ErrorContainer Prompt: Error Messages
      mask DialogControl ErrorText Prompt: The interpreted StateVar value is not yet available
      mask DialogControl TspPathText Prompt: TSP: Current parameter name: [AudiopilotLfNoiseMicOut]
      mask Display:
      | % retrieve icon definition
      | [path,w,h] = TargetStateVarMask.Icon();
      | 
      | % retrieve the block's pixel size
      | pos = get(gcbh,'position');
      | bw = pos(3) - pos(1);
      | bh = pos(4) - pos(2);
      | 
      | % draw centered icon
      | xAdj = bw/2 - w/2 + 5;
      | yAdj = bh/2 - h/2 + 4;
      | for i=1:length(path)
      | 	patch(path(i).x+xAdj, path(i).y+yAdj, path(i).rgb);
      | end
      | 
      | % show the top name or an X
      | if (exist('ok','var') && ok)
      | 	text(bw*0.5, bh*0.2, tspPath, 'horizontalAlignment', 'center');
      | 	patch(0,0,[1 1 1]);
      | 	patch(bw,bh,[1 1 1]);
      | else
      | 	tx=bw*0.03;
      | 	ty=bh*0.03;
      | 	patch([0 tx bw bw-tx], [ty 0 bh-ty bh], [1 0 0]);
      | 	patch([0 bw-tx bw tx], [bh-ty 0 ty bh], [1 0 0]);
      | end
  MusicOut : Subsystem  mask(Talaria Target State Variable){TriggerInit=[500 416 640 484], TspName=MusicOut, StateName=MusicOut, UseSameName=on, IfdefMacro=[]}
      mask prompts: TriggerInit "Hidden: MoveFcn redraw"; TspName "Name:"; StateName "Name of StateVar:"; UseSameName "Use same name for state variable and TSP"; IfdefMacro "Additional #ifdef macro to enable trigger capture:"
      mask help: The TargetStateVar block encapsultes a Target State Probe (TSP), a State Variable, and a Trivial Interpretation between them.
      mask init:
      | [ok,tspPath,activeStatePath] = TargetStateVarMask.Init(gcbh);
      settings: MoveFcn=TargetStateVarMask.CB_TriggerInit(gcbh);
      mask Help: See help for StateVar and TSP blocks
      mask Callback TriggerInit: TargetStateVarMask.CB_TriggerInit(gcbh);
      mask TypeOptions TspName: TSP/TspName
      mask TypeOptions StateName: StateVar/StateName
      mask Callback UseSameName: TargetStateVarMask.CB_UseSameName(gcbh);
      mask TypeOptions IfdefMacro: TSP/IfdefMacro
      mask DialogControl AdvancedPanel Prompt: Advanced
      mask DialogControl ConvertToFullInterpretation Prompt: Irreversible conversion to full interpretation
      mask DialogControl ConvertToFullInterpretation Callback: TargetStateVarMask.CB_ConvertToFullInterpretation(gcbh);
      mask DialogControl ErrorContainer Prompt: Error Messages
      mask DialogControl ErrorText Prompt: The interpreted StateVar value is not yet available
      mask DialogControl TspPathText Prompt: TSP: Current parameter name: [AudiopilotLfNoiseMusicOut]
      mask Display:
      | % retrieve icon definition
      | [path,w,h] = TargetStateVarMask.Icon();
      | 
      | % retrieve the block's pixel size
      | pos = get(gcbh,'position');
      | bw = pos(3) - pos(1);
      | bh = pos(4) - pos(2);
      | 
      | % draw centered icon
      | xAdj = bw/2 - w/2 + 5;
      | yAdj = bh/2 - h/2 + 4;
      | for i=1:length(path)
      | 	patch(path(i).x+xAdj, path(i).y+yAdj, path(i).rgb);
      | end
      | 
      | % show the top name or an X
      | if (exist('ok','var') && ok)
      | 	text(bw*0.5, bh*0.2, tspPath, 'horizontalAlignment', 'center');
      | 	patch(0,0,[1 1 1]);
      | 	patch(bw,bh,[1 1 1]);
      | else
      | 	tx=bw*0.03;
      | 	ty=bh*0.03;
      | 	patch([0 tx bw bw-tx], [ty 0 bh-ty bh], [1 0 0]);
      | 	patch([0 bw-tx bw tx], [bh-ty 0 ty bh], [1 0 0]);
      | end
  NoiseOut : Subsystem  mask(Talaria Target State Variable){TriggerInit=[335 466 475 534], TspName=NoiseOut, StateName=NoiseOut, UseSameName=on, IfdefMacro=[]}
      mask prompts: TriggerInit "Hidden: MoveFcn redraw"; TspName "Name:"; StateName "Name of StateVar:"; UseSameName "Use same name for state variable and TSP"; IfdefMacro "Additional #ifdef macro to enable trigger capture:"
      mask help: The TargetStateVar block encapsultes a Target State Probe (TSP), a State Variable, and a Trivial Interpretation between them.
      mask init:
      | [ok,tspPath,activeStatePath] = TargetStateVarMask.Init(gcbh);
      settings: MoveFcn=TargetStateVarMask.CB_TriggerInit(gcbh);
      mask Help: See help for StateVar and TSP blocks
      mask Callback TriggerInit: TargetStateVarMask.CB_TriggerInit(gcbh);
      mask TypeOptions TspName: TSP/TspName
      mask TypeOptions StateName: StateVar/StateName
      mask Callback UseSameName: TargetStateVarMask.CB_UseSameName(gcbh);
      mask TypeOptions IfdefMacro: TSP/IfdefMacro
      mask DialogControl AdvancedPanel Prompt: Advanced
      mask DialogControl ConvertToFullInterpretation Prompt: Irreversible conversion to full interpretation
      mask DialogControl ConvertToFullInterpretation Callback: TargetStateVarMask.CB_ConvertToFullInterpretation(gcbh);
      mask DialogControl ErrorContainer Prompt: Error Messages
      mask DialogControl ErrorText Prompt: The interpreted StateVar value is not yet available
      mask DialogControl TspPathText Prompt: TSP: Current parameter name: [AudiopilotLfNoiseNoiseOut]
      mask Display:
      | % retrieve icon definition
      | [path,w,h] = TargetStateVarMask.Icon();
      | 
      | % retrieve the block's pixel size
      | pos = get(gcbh,'position');
      | bw = pos(3) - pos(1);
      | bh = pos(4) - pos(2);
      | 
      | % draw centered icon
      | xAdj = bw/2 - w/2 + 5;
      | yAdj = bh/2 - h/2 + 4;
      | for i=1:length(path)
      | 	patch(path(i).x+xAdj, path(i).y+yAdj, path(i).rgb);
      | end
      | 
      | % show the top name or an X
      | if (exist('ok','var') && ok)
      | 	text(bw*0.5, bh*0.2, tspPath, 'horizontalAlignment', 'center');
      | 	patch(0,0,[1 1 1]);
      | 	patch(bw,bh,[1 1 1]);
      | else
      | 	tx=bw*0.03;
      | 	ty=bh*0.03;
      | 	patch([0 tx bw bw-tx], [ty 0 bh-ty bh], [1 0 0]);
      | 	patch([0 bw-tx bw tx], [bh-ty 0 ty bh], [1 0 0]);
      | end
  PostSlew : Subsystem  mask(Talaria Target State Variable){TriggerInit=[1020 201 1160 269], TspName=PostSlew, StateName=PostSlew, UseSameName=on, IfdefMacro=[]}
      mask prompts: TriggerInit "Hidden: MoveFcn redraw"; TspName "Name:"; StateName "Name of StateVar:"; UseSameName "Use same name for state variable and TSP"; IfdefMacro "Additional #ifdef macro to enable trigger capture:"
      mask help: The TargetStateVar block encapsultes a Target State Probe (TSP), a State Variable, and a Trivial Interpretation between them.
      mask init:
      | [ok,tspPath,activeStatePath] = TargetStateVarMask.Init(gcbh);
      settings: MoveFcn=TargetStateVarMask.CB_TriggerInit(gcbh);
      mask Help: See help for StateVar and TSP blocks
      mask Callback TriggerInit: TargetStateVarMask.CB_TriggerInit(gcbh);
      mask TypeOptions TspName: TSP/TspName
      mask TypeOptions StateName: StateVar/StateName
      mask Callback UseSameName: TargetStateVarMask.CB_UseSameName(gcbh);
      mask TypeOptions IfdefMacro: TSP/IfdefMacro
      mask DialogControl AdvancedPanel Prompt: Advanced
      mask DialogControl ConvertToFullInterpretation Prompt: Irreversible conversion to full interpretation
      mask DialogControl ConvertToFullInterpretation Callback: TargetStateVarMask.CB_ConvertToFullInterpretation(gcbh);
      mask DialogControl ErrorContainer Prompt: Error Messages
      mask DialogControl ErrorText Prompt: The interpreted StateVar value is not yet available
      mask DialogControl TspPathText Prompt: TSP: Current parameter name: [AudiopilotLfNoisePostSlew]
      mask Display:
      | % retrieve icon definition
      | [path,w,h] = TargetStateVarMask.Icon();
      | 
      | % retrieve the block's pixel size
      | pos = get(gcbh,'position');
      | bw = pos(3) - pos(1);
      | bh = pos(4) - pos(2);
      | 
      | % draw centered icon
      | xAdj = bw/2 - w/2 + 5;
      | yAdj = bh/2 - h/2 + 4;
      | for i=1:length(path)
      | 	patch(path(i).x+xAdj, path(i).y+yAdj, path(i).rgb);
      | end
      | 
      | % show the top name or an X
      | if (exist('ok','var') && ok)
      | 	text(bw*0.5, bh*0.2, tspPath, 'horizontalAlignment', 'center');
      | 	patch(0,0,[1 1 1]);
      | 	patch(bw,bh,[1 1 1]);
      | else
      | 	tx=bw*0.03;
      | 	ty=bh*0.03;
      | 	patch([0 tx bw bw-tx], [ty 0 bh-ty bh], [1 0 0]);
      | 	patch([0 bw-tx bw tx], [bh-ty 0 ty bh], [1 0 0]);
      | end
  PreSlew : Subsystem  mask(Talaria Target State Variable){TriggerInit=[1020 296 1160 364], TspName=PreSlew, StateName=PreSlew, UseSameName=on, IfdefMacro=[]}
      mask prompts: TriggerInit "Hidden: MoveFcn redraw"; TspName "Name:"; StateName "Name of StateVar:"; UseSameName "Use same name for state variable and TSP"; IfdefMacro "Additional #ifdef macro to enable trigger capture:"
      mask help: The TargetStateVar block encapsultes a Target State Probe (TSP), a State Variable, and a Trivial Interpretation between them.
      mask init:
      | [ok,tspPath,activeStatePath] = TargetStateVarMask.Init(gcbh);
      settings: MoveFcn=TargetStateVarMask.CB_TriggerInit(gcbh);
      mask Help: See help for StateVar and TSP blocks
      mask Callback TriggerInit: TargetStateVarMask.CB_TriggerInit(gcbh);
      mask TypeOptions TspName: TSP/TspName
      mask TypeOptions StateName: StateVar/StateName
      mask Callback UseSameName: TargetStateVarMask.CB_UseSameName(gcbh);
      mask TypeOptions IfdefMacro: TSP/IfdefMacro
      mask DialogControl AdvancedPanel Prompt: Advanced
      mask DialogControl ConvertToFullInterpretation Prompt: Irreversible conversion to full interpretation
      mask DialogControl ConvertToFullInterpretation Callback: TargetStateVarMask.CB_ConvertToFullInterpretation(gcbh);
      mask DialogControl ErrorContainer Prompt: Error Messages
      mask DialogControl ErrorText Prompt: The interpreted StateVar value is not yet available
      mask DialogControl TspPathText Prompt: TSP: Current parameter name: [AudiopilotLfNoisePreSlew]
      mask Display:
      | % retrieve icon definition
      | [path,w,h] = TargetStateVarMask.Icon();
      | 
      | % retrieve the block's pixel size
      | pos = get(gcbh,'position');
      | bw = pos(3) - pos(1);
      | bh = pos(4) - pos(2);
      | 
      | % draw centered icon
      | xAdj = bw/2 - w/2 + 5;
      | yAdj = bh/2 - h/2 + 4;
      | for i=1:length(path)
      | 	patch(path(i).x+xAdj, path(i).y+yAdj, path(i).rgb);
      | end
      | 
      | % show the top name or an X
      | if (exist('ok','var') && ok)
      | 	text(bw*0.5, bh*0.2, tspPath, 'horizontalAlignment', 'center');
      | 	patch(0,0,[1 1 1]);
      | 	patch(bw,bh,[1 1 1]);
      | else
      | 	tx=bw*0.03;
      | 	ty=bh*0.03;
      | 	patch([0 tx bw bw-tx], [ty 0 bh-ty bh], [1 0 0]);
      | 	patch([0 bw-tx bw tx], [bh-ty 0 ty bh], [1 0 0]);
      | end
  PreSpeedBound : Subsystem  mask(Talaria Target State Variable){TriggerInit=[1225 201 1365 269], TspName=PreSpeedBound, StateName=PreSpeedBound, UseSameName=on, IfdefMacro=[]}
      mask prompts: TriggerInit "Hidden: MoveFcn redraw"; TspName "Name:"; StateName "Name of StateVar:"; UseSameName "Use same name for state variable and TSP"; IfdefMacro "Additional #ifdef macro to enable trigger capture:"
      mask help: The TargetStateVar block encapsultes a Target State Probe (TSP), a State Variable, and a Trivial Interpretation between them.
      mask init:
      | [ok,tspPath,activeStatePath] = TargetStateVarMask.Init(gcbh);
      settings: MoveFcn=TargetStateVarMask.CB_TriggerInit(gcbh);
      mask Help: See help for StateVar and TSP blocks
      mask Callback TriggerInit: TargetStateVarMask.CB_TriggerInit(gcbh);
      mask TypeOptions TspName: TSP/TspName
      mask TypeOptions StateName: StateVar/StateName
      mask Callback UseSameName: TargetStateVarMask.CB_UseSameName(gcbh);
      mask TypeOptions IfdefMacro: TSP/IfdefMacro
      mask DialogControl AdvancedPanel Prompt: Advanced
      mask DialogControl ConvertToFullInterpretation Prompt: Irreversible conversion to full interpretation
      mask DialogControl ConvertToFullInterpretation Callback: TargetStateVarMask.CB_ConvertToFullInterpretation(gcbh);
      mask DialogControl ErrorContainer Prompt: Error Messages
      mask DialogControl ErrorText Prompt: The interpreted StateVar value is not yet available
      mask DialogControl TspPathText Prompt: TSP: Current parameter name: [AudiopilotLfNoisePreSpeedBound]
      mask Display:
      | % retrieve icon definition
      | [path,w,h] = TargetStateVarMask.Icon();
      | 
      | % retrieve the block's pixel size
      | pos = get(gcbh,'position');
      | bw = pos(3) - pos(1);
      | bh = pos(4) - pos(2);
      | 
      | % draw centered icon
      | xAdj = bw/2 - w/2 + 5;
      | yAdj = bh/2 - h/2 + 4;
      | for i=1:length(path)
      | 	patch(path(i).x+xAdj, path(i).y+yAdj, path(i).rgb);
      | end
      | 
      | % show the top name or an X
      | if (exist('ok','var') && ok)
      | 	text(bw*0.5, bh*0.2, tspPath, 'horizontalAlignment', 'center');
      | 	patch(0,0,[1 1 1]);
      | 	patch(bw,bh,[1 1 1]);
      | else
      | 	tx=bw*0.03;
      | 	ty=bh*0.03;
      | 	patch([0 tx bw bw-tx], [ty 0 bh-ty bh], [1 0 0]);
      | 	patch([0 bw-tx bw tx], [bh-ty 0 ty bh], [1 0 0]);
      | end
  SpeedBoundsAndNoiseSlew : Subsystem
